simulink model "Sim_Induct_Harmon"  (R2017b)
settings: Solver=FixedStepAuto  StartTime=0.0  StopTime=t_total  FixedStep=1e-6  MaxStep=1e-4  RelTol=1e-3
values from neighbouring files (symbols this model uses):
  C21 = 100e-6    (= 0.0001)    [main_simu.m]
  C22 = 100e-6    (= 0.0001)    [main_simu.m]
  C23 = 220e-6    (= 0.00022)    [main_simu.m]
  C24 = 330e-6    (= 0.00033)    [main_simu.m]
  L41 = 10e-3    (= 0.01)    [main_simu.m]
  L42 = 10e-3    (= 0.01)    [main_simu.m]
  L43 = 10e-3    (= 0.01)    [main_simu.m]
  L44 = 100e-3    (= 0.1)    [main_simu.m]
  L61 = 1e-3    (= 0.001)    [main_simu.m]
  L62 = 1e-3    (= 0.001)    [main_simu.m]
  L63 = 1e-3    (= 0.001)    [main_simu.m]
  L64 = 1e-3    (= 0.001)    [main_simu.m]
  R21 = 2e3    (= 2000)    [main_simu.m]
  R22 = 1e3    (= 1000)    [main_simu.m]
  R23 = 500    [main_simu.m]
  R24 = 300    [main_simu.m]
  R31 = 2.5    [main_simu.m]
  R32 = 5    [main_simu.m]
  R33 = 8    [main_simu.m]
  R34 = 10    [main_simu.m]
  R41 = 10    [main_simu.m]
  R42 = 20    [main_simu.m]
  R43 = 30    [main_simu.m]
  R44 = 30    [main_simu.m]
  R51 = 10    [main_simu.m]
  R52 = 12    [main_simu.m]
  R53 = 15    [main_simu.m]
  R54 = 20    [main_simu.m]
  R61 = 10    [main_simu.m]
  R62 = 5    [main_simu.m]
  R63 = 30    [main_simu.m]
  R64 = 105    [main_simu.m]
  R71 = 5    [main_simu.m]
  R72 = 10    [main_simu.m]
  R73 = 20    [main_simu.m]
  R74 = 50    [main_simu.m]
  sim_off = sim_on    [double.m]    (also in fourfold.m; individual.m; main_simu.m; quintuple.m)
  sim_on = 50*ones(1,28)    [double.m]    (also in fourfold.m; individual.m; main_simu.m = 50*ones(1,num_cargas); quintuple.m)
  Valpha5 = 60    [main_simu.m]
  Valpha6 = 60    [main_simu.m]
undefined symbols (not defined in the file or in its folder): J, Laq, Lse, R, Ra, Rse, SEIP4, SEVP4, wm0, wmo
libraries: powerlib x225, simulink x72
(part 2 of 3)

== system Sim_Induct_Harmon/ON_OFF_25 ==
  Clock8 : Clock
  Compare To Constant5 : simulink/Logic and Bit Operations/Compare To Constant  relop=>=  const=sim_on(25)  OutDataTypeStr=boolean
  Compare To Constat6 : simulink/Logic and Bit Operations/Compare To Constant  relop=<=  const=sim_off(25)  OutDataTypeStr=boolean
  OFF5 : powerlib/Power Electronics/Ideal Switch  Ron=0.001  Lon=0  IC=0  Rs=1e5  Cs=inf  Measurements=off
  ON5 : powerlib/Power Electronics/Ideal Switch  Ron=0.001  Lon=0  IC=0  Rs=1e5  Cs=inf  Measurements=off
  Conn1 : PMIOPort  Port=1  Side=Left
  Conn2 : PMIOPort  Port=2  Side=Right
  wires:
  Clock8/1 -> Compare To Constat6/1, Compare To Constant5/1
  Compare To Constat6/1 -> OFF5/1
  Compare To Constant5/1 -> ON5/1
  connections:
  ON5/RConn1 -- OFF5/LConn1
  OFF5/RConn1 -- Conn2/RConn1
  ON5/LConn1 -- Conn1/RConn1

== system Sim_Induct_Harmon/ON_OFF_26 ==
  Clock8 : Clock
  Compare To Constant5 : simulink/Logic and Bit Operations/Compare To Constant  relop=>=  const=sim_on(26)  OutDataTypeStr=boolean
  Compare To Constat6 : simulink/Logic and Bit Operations/Compare To Constant  relop=<=  const=sim_off(26)  OutDataTypeStr=boolean
  OFF5 : powerlib/Power Electronics/Ideal Switch  Ron=0.001  Lon=0  IC=0  Rs=1e5  Cs=inf  Measurements=off
  ON5 : powerlib/Power Electronics/Ideal Switch  Ron=0.001  Lon=0  IC=0  Rs=1e5  Cs=inf  Measurements=off
  Conn1 : PMIOPort  Port=1  Side=Left
  Conn2 : PMIOPort  Port=2  Side=Right
  wires:
  Clock8/1 -> Compare To Constat6/1, Compare To Constant5/1
  Compare To Constat6/1 -> OFF5/1
  Compare To Constant5/1 -> ON5/1
  connections:
  ON5/RConn1 -- OFF5/LConn1
  OFF5/RConn1 -- Conn2/RConn1
  ON5/LConn1 -- Conn1/RConn1

== system Sim_Induct_Harmon/ON_OFF_27 ==
  Clock8 : Clock
  Compare To Constant5 : simulink/Logic and Bit Operations/Compare To Constant  relop=>=  const=sim_on(27)  OutDataTypeStr=boolean
  Compare To Constat6 : simulink/Logic and Bit Operations/Compare To Constant  relop=<=  const=sim_off(27)  OutDataTypeStr=boolean
  OFF5 : powerlib/Power Electronics/Ideal Switch  Ron=0.001  Lon=0  IC=0  Rs=1e5  Cs=inf  Measurements=off
  ON5 : powerlib/Power Electronics/Ideal Switch  Ron=0.001  Lon=0  IC=0  Rs=1e5  Cs=inf  Measurements=off
  Conn1 : PMIOPort  Port=1  Side=Left
  Conn2 : PMIOPort  Port=2  Side=Right
  wires:
  Clock8/1 -> Compare To Constat6/1, Compare To Constant5/1
  Compare To Constat6/1 -> OFF5/1
  Compare To Constant5/1 -> ON5/1
  connections:
  ON5/RConn1 -- OFF5/LConn1
  OFF5/RConn1 -- Conn2/RConn1
  ON5/LConn1 -- Conn1/RConn1

== system Sim_Induct_Harmon/ON_OFF_28 ==
  Clock8 : Clock
  Compare To Constant5 : simulink/Logic and Bit Operations/Compare To Constant  relop=>=  const=sim_on(28)  OutDataTypeStr=boolean
  Compare To Constat6 : simulink/Logic and Bit Operations/Compare To Constant  relop=<=  const=sim_off(28)  OutDataTypeStr=boolean
  OFF5 : powerlib/Power Electronics/Ideal Switch  Ron=0.001  Lon=0  IC=0  Rs=1e5  Cs=inf  Measurements=off
  ON5 : powerlib/Power Electronics/Ideal Switch  Ron=0.001  Lon=0  IC=0  Rs=1e5  Cs=inf  Measurements=off
  Conn1 : PMIOPort  Port=1  Side=Left
  Conn2 : PMIOPort  Port=2  Side=Right
  wires:
  Clock8/1 -> Compare To Constat6/1, Compare To Constant5/1
  Compare To Constat6/1 -> OFF5/1
  Compare To Constant5/1 -> ON5/1
  connections:
  ON5/RConn1 -- OFF5/LConn1
  OFF5/RConn1 -- Conn2/RConn1
  ON5/LConn1 -- Conn1/RConn1

== system Sim_Induct_Harmon/ON_OFF_3 ==
  Clock1 : Clock
  Clock2 : Clock
  Clock3 : Clock
  Compare To Constant : simulink/Logic and Bit Operations/Compare To Constant  relop=>=  const=sim_on(3)  OutDataTypeStr=boolean
  Compare To Constant1 : simulink/Logic and Bit Operations/Compare To Constant  relop=>=  const=sim_off(3)  OutDataTypeStr=boolean
  Compare To Constant2 : simulink/Logic and Bit Operations/Compare To Constant  relop=>=  const=sim_on(3)  OutDataTypeStr=boolean
  Constant : Constant  Value=0
  Constant1 : Constant  Value=0
  Ideal Switch : powerlib/Power Electronics/Ideal Switch  Ron=0.001  Lon=0  IC=0  Rs=1e5  Cs=inf  Measurements=off
  Switch : Switch
  Switch1 : Switch
  Conn1 : PMIOPort  Port=1  Side=Left
  Conn2 : PMIOPort  Port=2  Side=Left
  tag scope: tensao_3=global
  wires:
  Switch1/1 -> [tensao_3]
  Constant/1 -> Switch/3
  Switch/1 -> Switch1/3
  Clock1/1 -> Compare To Constant/1
  Clock2/1 -> Compare To Constant1/1
  Compare To Constant1/1 -> Switch1/2
  [fonte_tensao] -> Switch/1
  Constant1/1 -> Switch1/1
  Compare To Constant/1 -> Switch/2
  Clock3/1 -> Compare To Constant2/1
  Compare To Constant2/1 -> Ideal Switch/1
  connections:
  Conn1/RConn1 -- Ideal Switch/LConn1
  Ideal Switch/RConn1 -- Conn2/RConn1

== system Sim_Induct_Harmon/ON_OFF_4 ==
  Clock1 : Clock
  Clock2 : Clock
  Clock3 : Clock
  Compare To Constant : simulink/Logic and Bit Operations/Compare To Constant  relop=>=  const=sim_on(4)  OutDataTypeStr=boolean
  Compare To Constant1 : simulink/Logic and Bit Operations/Compare To Constant  relop=>=  const=sim_off(4)  OutDataTypeStr=boolean
  Compare To Constant2 : simulink/Logic and Bit Operations/Compare To Constant  relop=>=  const=sim_on(4)  OutDataTypeStr=boolean
  Constant : Constant  Value=0
  Constant1 : Constant  Value=0
  Ideal Switch : powerlib/Power Electronics/Ideal Switch  Ron=0.001  Lon=0  IC=0  Rs=1e5  Cs=inf  Measurements=off
  Switch : Switch
  Switch1 : Switch
  Conn1 : PMIOPort  Port=1  Side=Left
  Conn2 : PMIOPort  Port=2  Side=Left
  tag scope: tensao_4=global
  wires:
  Switch1/1 -> [tensao_4]
  Constant/1 -> Switch/3
  Switch/1 -> Switch1/3
  Clock1/1 -> Compare To Constant/1
  Clock2/1 -> Compare To Constant1/1
  Compare To Constant1/1 -> Switch1/2
  [fonte_tensao] -> Switch/1
  Constant1/1 -> Switch1/1
  Compare To Constant/1 -> Switch/2
  Clock3/1 -> Compare To Constant2/1
  Compare To Constant2/1 -> Ideal Switch/1
  connections:
  Conn1/RConn1 -- Ideal Switch/LConn1
  Ideal Switch/RConn1 -- Conn2/RConn1

== system Sim_Induct_Harmon/ON_OFF_5 ==
  Clock1 : Clock
  Compare To Constant1 : simulink/Logic and Bit Operations/Compare To Constant  relop=>=  const=sim_on(5)  OutDataTypeStr=boolean
  Compare To Constat1 : simulink/Logic and Bit Operations/Compare To Constant  relop=<=  const=sim_off(5)  OutDataTypeStr=boolean
  OFF1 : powerlib/Power Electronics/Ideal Switch  Ron=0.001  Lon=0  IC=0  Rs=1e5  Cs=inf  Measurements=off
  ON1 : powerlib/Power Electronics/Ideal Switch  Ron=0.001  Lon=0  IC=0  Rs=1e5  Cs=inf  Measurements=off
  Conn1 : PMIOPort  Port=1  Side=Left
  Conn2 : PMIOPort  Port=2  Side=Right
  wires:
  Compare To Constat1/1 -> OFF1/1
  Compare To Constant1/1 -> ON1/1
  Clock1/1 -> Compare To Constat1/1, Compare To Constant1/1
  connections:
  ON1/RConn1 -- OFF1/LConn1
  Conn1/RConn1 -- ON1/LConn1
  OFF1/RConn1 -- Conn2/RConn1

== system Sim_Induct_Harmon/ON_OFF_6 ==
  Clock1 : Clock
  Compare To Constant1 : simulink/Logic and Bit Operations/Compare To Constant  relop=>=  const=sim_on(6)  OutDataTypeStr=boolean
  Compare To Constat1 : simulink/Logic and Bit Operations/Compare To Constant  relop=<=  const=sim_off(6)  OutDataTypeStr=boolean
  OFF1 : powerlib/Power Electronics/Ideal Switch  Ron=0.001  Lon=0  IC=0  Rs=1e5  Cs=inf  Measurements=off
  ON1 : powerlib/Power Electronics/Ideal Switch  Ron=0.001  Lon=0  IC=0  Rs=1e5  Cs=inf  Measurements=off
  Conn1 : PMIOPort  Port=1  Side=Left
  Conn2 : PMIOPort  Port=2  Side=Right
  wires:
  Compare To Constat1/1 -> OFF1/1
  Compare To Constant1/1 -> ON1/1
  Clock1/1 -> Compare To Constat1/1, Compare To Constant1/1
  connections:
  ON1/RConn1 -- OFF1/LConn1
  Conn1/RConn1 -- ON1/LConn1
  OFF1/RConn1 -- Conn2/RConn1

== system Sim_Induct_Harmon/ON_OFF_7 ==
  Clock1 : Clock
  Compare To Constant1 : simulink/Logic and Bit Operations/Compare To Constant  relop=>=  const=sim_on(7)  OutDataTypeStr=boolean
  Compare To Constat1 : simulink/Logic and Bit Operations/Compare To Constant  relop=<=  const=sim_off(7)  OutDataTypeStr=boolean
  OFF1 : powerlib/Power Electronics/Ideal Switch  Ron=0.001  Lon=0  IC=0  Rs=1e5  Cs=inf  Measurements=off
  ON1 : powerlib/Power Electronics/Ideal Switch  Ron=0.001  Lon=0  IC=0  Rs=1e5  Cs=inf  Measurements=off
  Conn1 : PMIOPort  Port=1  Side=Left
  Conn2 : PMIOPort  Port=2  Side=Right
  wires:
  Compare To Constat1/1 -> OFF1/1
  Compare To Constant1/1 -> ON1/1
  Clock1/1 -> Compare To Constat1/1, Compare To Constant1/1
  connections:
  ON1/RConn1 -- OFF1/LConn1
  Conn1/RConn1 -- ON1/LConn1
  OFF1/RConn1 -- Conn2/RConn1

== system Sim_Induct_Harmon/ON_OFF_8 ==
  Clock1 : Clock
  Compare To Constant1 : simulink/Logic and Bit Operations/Compare To Constant  relop=>=  const=sim_on(8)  OutDataTypeStr=boolean
  Compare To Constat1 : simulink/Logic and Bit Operations/Compare To Constant  relop=<=  const=sim_off(8)  OutDataTypeStr=boolean
  OFF1 : powerlib/Power Electronics/Ideal Switch  Ron=0.001  Lon=0  IC=0  Rs=1e5  Cs=inf  Measurements=off
  ON1 : powerlib/Power Electronics/Ideal Switch  Ron=0.001  Lon=0  IC=0  Rs=1e5  Cs=inf  Measurements=off
  Conn1 : PMIOPort  Port=1  Side=Left
  Conn2 : PMIOPort  Port=2  Side=Right
  wires:
  Compare To Constat1/1 -> OFF1/1
  Compare To Constant1/1 -> ON1/1
  Clock1/1 -> Compare To Constat1/1, Compare To Constant1/1
  connections:
  ON1/RConn1 -- OFF1/LConn1
  Conn1/RConn1 -- ON1/LConn1
  OFF1/RConn1 -- Conn2/RConn1

== system Sim_Induct_Harmon/ON_OFF_9 ==
  Clock4 : Clock
  Compare To Constant2 : simulink/Logic and Bit Operations/Compare To Constant  relop=>=  const=sim_on(9)  OutDataTypeStr=boolean
  Compare To Constat3 : simulink/Logic and Bit Operations/Compare To Constant  relop=<=  const=sim_off(9)  OutDataTypeStr=boolean
  OFF2 : powerlib/Power Electronics/Ideal Switch  Ron=0.001  Lon=0  IC=0  Rs=1e5  Cs=inf  Measurements=off
  ON2 : powerlib/Power Electronics/Ideal Switch  Ron=0.001  Lon=0  IC=0  Rs=1e5  Cs=inf  Measurements=off
  Conn1 : PMIOPort  Port=1  Side=Left
  Conn2 : PMIOPort  Port=2  Side=Right
  wires:
  Compare To Constant2/1 -> ON2/1
  Compare To Constat3/1 -> OFF2/1
  Clock4/1 -> Compare To Constat3/1, Compare To Constant2/1
  connections:
  OFF2/RConn1 -- Conn2/RConn1
  ON2/RConn1 -- OFF2/LConn1
  ON2/LConn1 -- Conn1/RConn1

== system Sim_Induct_Harmon/PONTE_DIODO_1 ==
  Diode{,1..3} (4 alike) : powerlib/Power Electronics/Diode  Ron=0.001  Lon=0  Vf=0.8  IC=0  UseSnubber=0  Rs=500  Cs=250e-9  Measurements=off
  Scope : Scope
  Scope1 : Scope
  Series RLC Branch : powerlib/Elements/Series RLC Branch  LConnTagsString=__new0  RConnTagsString=__new0  BranchType=C  Resistance=R  Inductance=1e-3  SetiL0=off  InitialCurrent=0  Capacitance=C21  Setx0=off  InitialVoltage=0  Measurements=None
  Series RLC Branch1 : powerlib/Elements/Series RLC Branch  LConnTagsString=__new0  RConnTagsString=__new0  BranchType=R  Resistance=R21  Inductance=1e-3  SetiL0=off  InitialCurrent=0  Capacitance=1e-6  Setx0=off  InitialVoltage=0  Measurements=None
  Series RLC Branch2 : powerlib/Elements/Series RLC Branch  LConnTagsString=__new0  RConnTagsString=__new0  BranchType=R  Resistance=10  Inductance=1e-3  SetiL0=off  InitialCurrent=0  Capacitance=C21  Setx0=off  InitialVoltage=0  Measurements=None
  To Workspace1 : ToWorkspace  VariableName=corrente_ponte_1  SampleTime=-1
  To Workspace4 : ToWorkspace  VariableName=tensao_ponte_1  SampleTime=-1
  V_Load : powerlib/Measurements/Voltage Measurement  PhasorSimulation=off  OutputType=Complex  PSBequivalent=0
  i_Load : powerlib/Measurements/Current Measurement  Tag=PoWeRsYsTeMmEaSuReMeNt  PhasorSimulation=off  OutputType=Magnitude  PSBequivalent=0
  Conn1 : PMIOPort  Port=1  Side=Left
  Conn2 : PMIOPort  Port=2  Side=Left
  wires:
  i_Load/1 -> To Workspace1/1, Scope1/1
  V_Load/1 -> To Workspace4/1, Scope/1
  connections:
  Conn1/RConn1 -- i_Load/LConn1
  Diode1/LConn1 -- Conn2/RConn1 -- Diode3/RConn1
  Series RLC Branch/LConn1 -- Diode/RConn1 -- Diode1/RConn1 -- V_Load/LConn1 -- Series RLC Branch1/LConn1
  Series RLC Branch/RConn1 -- Diode2/LConn1 -- Diode3/LConn1 -- V_Load/LConn2 -- Series RLC Branch1/RConn1
  Series RLC Branch2/RConn1 -- Diode2/RConn1 -- Diode/LConn1
  i_Load/RConn1 -- Series RLC Branch2/LConn1

== system Sim_Induct_Harmon/PONTE_DIODO_2 ==
  Diode{,1..3} (4 alike) : powerlib/Power Electronics/Diode  Ron=0.001  Lon=0  Vf=0.8  IC=0  UseSnubber=0  Rs=500  Cs=250e-9  Measurements=off
  Scope : Scope
  Scope1 : Scope
  Series RLC Branch : powerlib/Elements/Series RLC Branch  LConnTagsString=__new0  RConnTagsString=__new0  BranchType=C  Resistance=R  Inductance=1e-3  SetiL0=off  InitialCurrent=0  Capacitance=C22  Setx0=off  InitialVoltage=0  Measurements=None
  Series RLC Branch1 : powerlib/Elements/Series RLC Branch  LConnTagsString=__new0  RConnTagsString=__new0  BranchType=R  Resistance=R22  Inductance=1e-3  SetiL0=off  InitialCurrent=0  Capacitance=1e-6  Setx0=off  InitialVoltage=0  Measurements=None
  Series RLC Branch2 : powerlib/Elements/Series RLC Branch  LConnTagsString=__new0  RConnTagsString=__new0  BranchType=R  Resistance=10  Inductance=1e-3  SetiL0=off  InitialCurrent=0  Capacitance=C21  Setx0=off  InitialVoltage=0  Measurements=None
  To Workspace1 : ToWorkspace  VariableName=corrente_ponte_2  SampleTime=-1
  To Workspace4 : ToWorkspace  VariableName=tensao_ponte_2  SampleTime=-1
  V_Load : powerlib/Measurements/Voltage Measurement  PhasorSimulation=off  OutputType=Complex  PSBequivalent=0
  i_Load : powerlib/Measurements/Current Measurement  Tag=PoWeRsYsTeMmEaSuReMeNt  PhasorSimulation=off  OutputType=Magnitude  PSBequivalent=0
  Conn1 : PMIOPort  Port=1  Side=Left
  Conn2 : PMIOPort  Port=2  Side=Left
  wires:
  i_Load/1 -> To Workspace1/1, Scope1/1
  V_Load/1 -> To Workspace4/1, Scope/1
  connections:
  Conn1/RConn1 -- i_Load/LConn1
  Diode1/LConn1 -- Conn2/RConn1 -- Diode3/RConn1
  Series RLC Branch/LConn1 -- Diode/RConn1 -- Diode1/RConn1 -- V_Load/LConn1 -- Series RLC Branch1/LConn1
  Series RLC Branch/RConn1 -- Diode2/LConn1 -- Diode3/LConn1 -- V_Load/LConn2 -- Series RLC Branch1/RConn1
  Diode2/RConn1 -- Series RLC Branch2/RConn1 -- Diode/LConn1
  i_Load/RConn1 -- Series RLC Branch2/LConn1

== system Sim_Induct_Harmon/PONTE_DIODO_3 ==
  Diode{,1..3} (4 alike) : powerlib/Power Electronics/Diode  Ron=0.001  Lon=0  Vf=0.8  IC=0  UseSnubber=0  Rs=500  Cs=250e-9  Measurements=off
  Scope : Scope
  Scope1 : Scope
  Series RLC Branch : powerlib/Elements/Series RLC Branch  LConnTagsString=__new0  RConnTagsString=__new0  BranchType=C  Resistance=R  Inductance=1e-3  SetiL0=off  InitialCurrent=0  Capacitance=C23  Setx0=off  InitialVoltage=0  Measurements=None
  Series RLC Branch1 : powerlib/Elements/Series RLC Branch  LConnTagsString=__new0  RConnTagsString=__new0  BranchType=R  Resistance=R23  Inductance=1e-3  SetiL0=off  InitialCurrent=0  Capacitance=1e-6  Setx0=off  InitialVoltage=0  Measurements=None
  Series RLC Branch2 : powerlib/Elements/Series RLC Branch  LConnTagsString=__new0  RConnTagsString=__new0  BranchType=R  Resistance=10  Inductance=1e-3  SetiL0=off  InitialCurrent=0  Capacitance=C21  Setx0=off  InitialVoltage=0  Measurements=None
  To Workspace1 : ToWorkspace  VariableName=corrente_ponte_3  SampleTime=-1
  To Workspace4 : ToWorkspace  VariableName=tensao_ponte_3  SampleTime=-1
  V_Load : powerlib/Measurements/Voltage Measurement  PhasorSimulation=off  OutputType=Complex  PSBequivalent=0
  i_Load : powerlib/Measurements/Current Measurement  Tag=PoWeRsYsTeMmEaSuReMeNt  PhasorSimulation=off  OutputType=Magnitude  PSBequivalent=0
  powergui : powerlib/powergui  Priority=1  SimulationMode=Discrete  SampleTime=1e-6  frequency=60  Iterations=100  frequencyindice=60  Pbase=100e6  ErrMax=1e-4  UnitsV=kV  UnitsW=MW  buscounter=0  FunctionMessages=off  echomessages=off  EnableUseOfTLC=off  CurrentSourceSwitches=off  DisableSnubberDevices=off  DisableRonSwitches=off  DisableVfSwitches=off  DisplayEquations=off  SolverType=Tustin/Backward Euler (TBE)  Interpol=off  ExternalGateDelay=off  methode=off  Ts=100  x0status=zero  SPID=off  SwTol=0  HookPort=off  RestoreLinks=warning  ResistiveCurrentMeasurement=off  Frange=[0:2:500]  Ylog=off  Xlog=on  ShowGrid=off  save=off  variable=ZData  structure=0  ZoomFFT=off  StartTime=0.0  cycles=1  DisplayStyle=1  fundamental=60  FreqAxis=off  MaxFrequency=1000  frequencyindicesteady=1  RmsSteady=1  display=off
  Conn1 : PMIOPort  Port=1  Side=Left
  Conn2 : PMIOPort  Port=2  Side=Left
  wires:
  i_Load/1 -> To Workspace1/1, Scope1/1
  V_Load/1 -> To Workspace4/1, Scope/1
  connections:
  Conn1/RConn1 -- i_Load/LConn1
  Diode1/LConn1 -- Conn2/RConn1 -- Diode3/RConn1
  Series RLC Branch/LConn1 -- Diode/RConn1 -- Diode1/RConn1 -- V_Load/LConn1 -- Series RLC Branch1/LConn1
  Series RLC Branch/RConn1 -- Diode2/LConn1 -- Diode3/LConn1 -- V_Load/LConn2 -- Series RLC Branch1/RConn1
  Diode/LConn1 -- Series RLC Branch2/RConn1 -- Diode2/RConn1
  i_Load/RConn1 -- Series RLC Branch2/LConn1

== system Sim_Induct_Harmon/PONTE_DIODO_4 ==
  Diode{,1..3} (4 alike) : powerlib/Power Electronics/Diode  Ron=0.001  Lon=0  Vf=0.8  IC=0  UseSnubber=0  Rs=500  Cs=250e-9  Measurements=off
  Scope : Scope
  Scope1 : Scope
  Series RLC Branch : powerlib/Elements/Series RLC Branch  LConnTagsString=__new0  RConnTagsString=__new0  BranchType=C  Resistance=R  Inductance=1e-3  SetiL0=off  InitialCurrent=0  Capacitance=C24  Setx0=off  InitialVoltage=0  Measurements=None
  Series RLC Branch1 : powerlib/Elements/Series RLC Branch  LConnTagsString=__new0  RConnTagsString=__new0  BranchType=R  Resistance=R24  Inductance=1e-3  SetiL0=off  InitialCurrent=0  Capacitance=1e-6  Setx0=off  InitialVoltage=0  Measurements=None
  Series RLC Branch2 : powerlib/Elements/Series RLC Branch  LConnTagsString=__new0  RConnTagsString=__new0  BranchType=R  Resistance=10  Inductance=1e-3  SetiL0=off  InitialCurrent=0  Capacitance=C21  Setx0=off  InitialVoltage=0  Measurements=None
  To Workspace1 : ToWorkspace  VariableName=corrente_ponte_4  SampleTime=-1
  To Workspace4 : ToWorkspace  VariableName=tensao_ponte_4  SampleTime=-1
  V_Load : powerlib/Measurements/Voltage Measurement  PhasorSimulation=off  OutputType=Complex  PSBequivalent=0
  i_Load : powerlib/Measurements/Current Measurement  Tag=PoWeRsYsTeMmEaSuReMeNt  PhasorSimulation=off  OutputType=Magnitude  PSBequivalent=0
  Conn1 : PMIOPort  Port=1  Side=Left
  Conn2 : PMIOPort  Port=2  Side=Left
  wires:
  i_Load/1 -> To Workspace1/1, Scope1/1
  V_Load/1 -> To Workspace4/1, Scope/1
  connections:
  Conn1/RConn1 -- i_Load/LConn1
  Diode1/LConn1 -- Conn2/RConn1 -- Diode3/RConn1
  Series RLC Branch/LConn1 -- Diode/RConn1 -- Diode1/RConn1 -- V_Load/LConn1 -- Series RLC Branch1/LConn1
  Series RLC Branch/RConn1 -- Diode2/LConn1 -- Diode3/LConn1 -- V_Load/LConn2 -- Series RLC Branch1/RConn1
  Diode/LConn1 -- Series RLC Branch2/RConn1 -- Diode2/RConn1
  i_Load/RConn1 -- Series RLC Branch2/LConn1

== system Sim_Induct_Harmon/RL_1 ==
  note: LOAD
  Scope : Scope
  Scope1 : Scope
  Series RLC Branch : powerlib/Elements/Series RLC Branch  LConnTagsString=__new0  RConnTagsString=__new0  BranchType=R  Resistance=R41  Inductance=1e-3  SetiL0=off  InitialCurrent=0  Capacitance=1e-6  Setx0=off  InitialVoltage=0  Measurements=None
  Series RLC Branch1 : powerlib/Elements/Series RLC Branch  LConnTagsString=__new0  RConnTagsString=__new0  BranchType=L  Resistance=1  Inductance=L41  SetiL0=off  InitialCurrent=0  Capacitance=1e-6  Setx0=off  InitialVoltage=0  Measurements=None
  To Workspace1 : ToWorkspace  VariableName=corrente_rl_1  SampleTime=-1
  To Workspace4 : ToWorkspace  VariableName=tensao_rl_1  SampleTime=-1
  V_Load : powerlib/Measurements/Voltage Measurement  PhasorSimulation=off  OutputType=Complex  PSBequivalent=0
  i_Load : powerlib/Measurements/Current Measurement  Tag=PoWeRsYsTeMmEaSuReMeNt  PhasorSimulation=off  OutputType=Magnitude  PSBequivalent=0
  Conn1 : PMIOPort  Port=1  Side=Left
  Conn2 : PMIOPort  Port=2  Side=Left
  wires:
  V_Load/1 -> To Workspace4/1, Scope/1
  i_Load/1 -> To Workspace1/1, Scope1/1
  connections:
  Series RLC Branch/LConn1 -- V_Load/LConn1 -- i_Load/RConn1
  Conn1/RConn1 -- i_Load/LConn1
  V_Load/LConn2 -- Conn2/RConn1 -- Series RLC Branch1/RConn1
  Series RLC Branch1/LConn1 -- Series RLC Branch/RConn1

== system Sim_Induct_Harmon/RL_2 ==
  note: LOAD
  Scope : Scope
  Scope1 : Scope
  Series RLC Branch : powerlib/Elements/Series RLC Branch  LConnTagsString=__new0  RConnTagsString=__new0  BranchType=R  Resistance=R42  Inductance=1e-3  SetiL0=off  InitialCurrent=0  Capacitance=1e-6  Setx0=off  InitialVoltage=0  Measurements=None
  Series RLC Branch1 : powerlib/Elements/Series RLC Branch  LConnTagsString=__new0  RConnTagsString=__new0  BranchType=L  Resistance=1  Inductance=L42  SetiL0=off  InitialCurrent=0  Capacitance=1e-6  Setx0=off  InitialVoltage=0  Measurements=None
  To Workspace1 : ToWorkspace  VariableName=corrente_rl_2  SampleTime=-1
  To Workspace4 : ToWorkspace  VariableName=tensao_rl_2  SampleTime=-1
  V_Load : powerlib/Measurements/Voltage Measurement  PhasorSimulation=off  OutputType=Complex  PSBequivalent=0
  i_Load : powerlib/Measurements/Current Measurement  Tag=PoWeRsYsTeMmEaSuReMeNt  PhasorSimulation=off  OutputType=Magnitude  PSBequivalent=0
  Conn1 : PMIOPort  Port=1  Side=Left
  Conn2 : PMIOPort  Port=2  Side=Left
  wires:
  V_Load/1 -> To Workspace4/1, Scope/1
  i_Load/1 -> To Workspace1/1, Scope1/1
  connections:
  Series RLC Branch/LConn1 -- V_Load/LConn1 -- i_Load/RConn1
  Conn1/RConn1 -- i_Load/LConn1
  V_Load/LConn2 -- Conn2/RConn1 -- Series RLC Branch1/RConn1
  Series RLC Branch1/LConn1 -- Series RLC Branch/RConn1

== system Sim_Induct_Harmon/RL_3 ==
  note: LOAD
  Scope : Scope
  Scope1 : Scope
  Series RLC Branch : powerlib/Elements/Series RLC Branch  LConnTagsString=__new0  RConnTagsString=__new0  BranchType=R  Resistance=R43  Inductance=1e-3  SetiL0=off  InitialCurrent=0  Capacitance=1e-6  Setx0=off  InitialVoltage=0  Measurements=None
  Series RLC Branch1 : powerlib/Elements/Series RLC Branch  LConnTagsString=__new0  RConnTagsString=__new0  BranchType=L  Resistance=1  Inductance=L43  SetiL0=off  InitialCurrent=0  Capacitance=1e-6  Setx0=off  InitialVoltage=0  Measurements=None
  To Workspace1 : ToWorkspace  VariableName=corrente_rl_3  SampleTime=-1
  To Workspace4 : ToWorkspace  VariableName=tensao_rl_3  SampleTime=-1
  V_Load : powerlib/Measurements/Voltage Measurement  PhasorSimulation=off  OutputType=Complex  PSBequivalent=0
  i_Load : powerlib/Measurements/Current Measurement  Tag=PoWeRsYsTeMmEaSuReMeNt  PhasorSimulation=off  OutputType=Magnitude  PSBequivalent=0
  Conn1 : PMIOPort  Port=1  Side=Left
  Conn2 : PMIOPort  Port=2  Side=Left
  wires:
  V_Load/1 -> To Workspace4/1, Scope/1
  i_Load/1 -> To Workspace1/1, Scope1/1
  connections:
  Series RLC Branch/LConn1 -- V_Load/LConn1 -- i_Load/RConn1
  Conn1/RConn1 -- i_Load/LConn1
  V_Load/LConn2 -- Conn2/RConn1 -- Series RLC Branch1/RConn1
  Series RLC Branch1/LConn1 -- Series RLC Branch/RConn1

== system Sim_Induct_Harmon/RL_4 ==
  note: LOAD
  Scope : Scope
  Scope1 : Scope
  Series RLC Branch : powerlib/Elements/Series RLC Branch  LConnTagsString=__new0  RConnTagsString=__new0  BranchType=R  Resistance=R44  Inductance=1e-3  SetiL0=off  InitialCurrent=0  Capacitance=1e-6  Setx0=off  InitialVoltage=0  Measurements=None
  Series RLC Branch1 : powerlib/Elements/Series RLC Branch  LConnTagsString=__new0  RConnTagsString=__new0  BranchType=L  Resistance=1  Inductance=L44  SetiL0=off  InitialCurrent=0  Capacitance=1e-6  Setx0=off  InitialVoltage=0  Measurements=None
  To Workspace1 : ToWorkspace  VariableName=corrente_rl_4  SampleTime=-1
  To Workspace4 : ToWorkspace  VariableName=tensao_rl_4  SampleTime=-1
  V_Load : powerlib/Measurements/Voltage Measurement  PhasorSimulation=off  OutputType=Complex  PSBequivalent=0
  i_Load : powerlib/Measurements/Current Measurement  Tag=PoWeRsYsTeMmEaSuReMeNt  PhasorSimulation=off  OutputType=Magnitude  PSBequivalent=0
  Conn1 : PMIOPort  Port=1  Side=Left
  Conn2 : PMIOPort  Port=2  Side=Left
  wires:
  V_Load/1 -> To Workspace4/1, Scope/1
  i_Load/1 -> To Workspace1/1, Scope1/1
  connections:
  Series RLC Branch/LConn1 -- V_Load/LConn1 -- i_Load/RConn1
  Conn1/RConn1 -- i_Load/LConn1
  V_Load/LConn2 -- Conn2/RConn1 -- Series RLC Branch1/RConn1
  Series RLC Branch1/LConn1 -- Series RLC Branch/RConn1

== system Sim_Induct_Harmon/R_1 ==
  note: LOAD
  Scope : Scope
  Scope1 : Scope
  Series RLC Branch : powerlib/Elements/Series RLC Branch  LConnTagsString=__new0  RConnTagsString=__new0  BranchType=R  Resistance=R31  Inductance=1e-3  SetiL0=off  InitialCurrent=0  Capacitance=1e-6  Setx0=off  InitialVoltage=0  Measurements=None
  To Workspace1 : ToWorkspace  VariableName=corrente_r_1  SampleTime=-1
  To Workspace4 : ToWorkspace  VariableName=tensao_r_1  SampleTime=-1
  V_Load : powerlib/Measurements/Voltage Measurement  PhasorSimulation=off  OutputType=Complex  PSBequivalent=0
  i_Load : powerlib/Measurements/Current Measurement  Tag=PoWeRsYsTeMmEaSuReMeNt  PhasorSimulation=off  OutputType=Magnitude  PSBequivalent=0
  Conn1 : PMIOPort  Port=1  Side=Left
  Conn2 : PMIOPort  Port=2  Side=Left
  wires:
  V_Load/1 -> To Workspace4/1, Scope/1
  i_Load/1 -> To Workspace1/1, Scope1/1
  connections:
  Series RLC Branch/LConn1 -- V_Load/LConn1 -- i_Load/RConn1
  Series RLC Branch/RConn1 -- V_Load/LConn2 -- Conn2/RConn1
  Conn1/RConn1 -- i_Load/LConn1

== system Sim_Induct_Harmon/R_2 ==
  note: LOAD
  Scope : Scope
  Scope1 : Scope
  Series RLC Branch : powerlib/Elements/Series RLC Branch  LConnTagsString=__new0  RConnTagsString=__new0  BranchType=R  Resistance=R32  Inductance=1e-3  SetiL0=off  InitialCurrent=0  Capacitance=1e-6  Setx0=off  InitialVoltage=0  Measurements=None
  To Workspace1 : ToWorkspace  VariableName=corrente_r_2  SampleTime=-1
  To Workspace4 : ToWorkspace  VariableName=tensao_r_2  SampleTime=-1
  V_Load : powerlib/Measurements/Voltage Measurement  PhasorSimulation=off  OutputType=Complex  PSBequivalent=0
  i_Load : powerlib/Measurements/Current Measurement  Tag=PoWeRsYsTeMmEaSuReMeNt  PhasorSimulation=off  OutputType=Magnitude  PSBequivalent=0
  Conn1 : PMIOPort  Port=1  Side=Left
  Conn2 : PMIOPort  Port=2  Side=Left
  wires:
  V_Load/1 -> To Workspace4/1, Scope/1
  i_Load/1 -> To Workspace1/1, Scope1/1
  connections:
  Series RLC Branch/LConn1 -- V_Load/LConn1 -- i_Load/RConn1
  Series RLC Branch/RConn1 -- V_Load/LConn2 -- Conn2/RConn1
  Conn1/RConn1 -- i_Load/LConn1

== system Sim_Induct_Harmon/R_3 ==
  note: LOAD
  Scope : Scope
  Scope1 : Scope
  Series RLC Branch : powerlib/Elements/Series RLC Branch  LConnTagsString=__new0  RConnTagsString=__new0  BranchType=R  Resistance=R33  Inductance=1e-3  SetiL0=off  InitialCurrent=0  Capacitance=1e-6  Setx0=off  InitialVoltage=0  Measurements=None
  To Workspace1 : ToWorkspace  VariableName=corrente_r_3  SampleTime=-1
  To Workspace4 : ToWorkspace  VariableName=tensao_r_3  SampleTime=-1
  V_Load : powerlib/Measurements/Voltage Measurement  PhasorSimulation=off  OutputType=Complex  PSBequivalent=0
  i_Load : powerlib/Measurements/Current Measurement  Tag=PoWeRsYsTeMmEaSuReMeNt  PhasorSimulation=off  OutputType=Magnitude  PSBequivalent=0
  Conn1 : PMIOPort  Port=1  Side=Left
  Conn2 : PMIOPort  Port=2  Side=Left
  wires:
  V_Load/1 -> To Workspace4/1, Scope/1
  i_Load/1 -> To Workspace1/1, Scope1/1
  connections:
  Series RLC Branch/LConn1 -- V_Load/LConn1 -- i_Load/RConn1
  Series RLC Branch/RConn1 -- V_Load/LConn2 -- Conn2/RConn1
  Conn1/RConn1 -- i_Load/LConn1

== system Sim_Induct_Harmon/R_4 ==
  note: LOAD
  Scope : Scope
  Scope1 : Scope
  Series RLC Branch : powerlib/Elements/Series RLC Branch  LConnTagsString=__new0  RConnTagsString=__new0  BranchType=R  Resistance=R34  Inductance=1e-3  SetiL0=off  InitialCurrent=0  Capacitance=1e-6  Setx0=off  InitialVoltage=0  Measurements=None
  To Workspace1 : ToWorkspace  VariableName=corrente_r_4  SampleTime=-1
  To Workspace4 : ToWorkspace  VariableName=tensao_r_4  SampleTime=-1
  V_Load : powerlib/Measurements/Voltage Measurement  PhasorSimulation=off  OutputType=Complex  PSBequivalent=0
  i_Load : powerlib/Measurements/Current Measurement  Tag=PoWeRsYsTeMmEaSuReMeNt  PhasorSimulation=off  OutputType=Magnitude  PSBequivalent=0
  Conn1 : PMIOPort  Port=1  Side=Left
  Conn2 : PMIOPort  Port=2  Side=Left
  wires:
  V_Load/1 -> To Workspace4/1, Scope/1
  i_Load/1 -> To Workspace1/1, Scope1/1
  connections:
  Series RLC Branch/LConn1 -- V_Load/LConn1 -- i_Load/RConn1
  Series RLC Branch/RConn1 -- V_Load/LConn2 -- Conn2/RConn1
  Conn1/RConn1 -- i_Load/LConn1

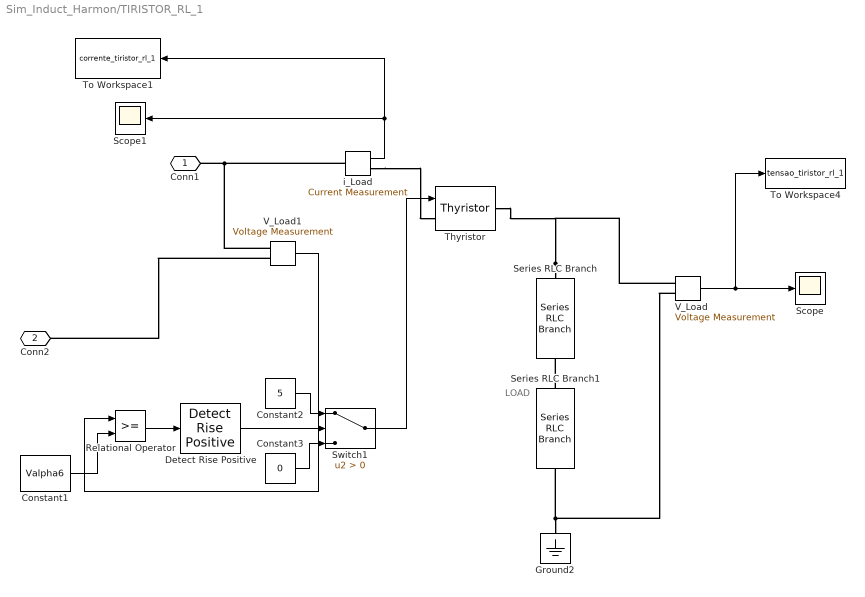
== system Sim_Induct_Harmon/TIRISTOR_RL_1 ==
  note: LOAD
  Constant1 : Constant  Value=Valpha6
  Constant2 : Constant  Value=5
  Constant3 : Constant  Value=0
  Detect Rise Positive : simulink/Logic and Bit Operations/Detect Rise Positive  vinit=0  OutDataTypeStr=boolean
  Ground2 : powerlib/Elements/Ground  LConnTagsString=a
  Relational Operator : RelationalOperator  OutDataTypeStr=boolean  RndMeth=Simplest
  Scope : Scope
  Scope1 : Scope
  Series RLC Branch : powerlib/Elements/Series RLC Branch  LConnTagsString=__new0  RConnTagsString=__new0  BranchType=R  Resistance=R61  Inductance=1e-3  SetiL0=off  InitialCurrent=0  Capacitance=1e-6  Setx0=off  InitialVoltage=0  Measurements=None
  Series RLC Branch1 : powerlib/Elements/Series RLC Branch  LConnTagsString=__new0  RConnTagsString=__new0  BranchType=L  Resistance=1  Inductance=L61  SetiL0=off  InitialCurrent=0  Capacitance=1e-6  Setx0=off  InitialVoltage=0  Measurements=None
  Switch1 : Switch  Criteria=u2 > Threshold
  Thyristor : powerlib/Power Electronics/Thyristor  Ron=0.001  Lon=0  Vf=0.8  IC=0  Rs=500  Cs=250e-9  Measurements=off
  To Workspace1 : ToWorkspace  VariableName=corrente_tiristor_rl_1  SampleTime=-1
  To Workspace4 : ToWorkspace  VariableName=tensao_tiristor_rl_1  SampleTime=-1
  V_Load : powerlib/Measurements/Voltage Measurement  PhasorSimulation=off  OutputType=Complex  PSBequivalent=0
  V_Load1 : powerlib/Measurements/Voltage Measurement  PhasorSimulation=off  OutputType=Complex  PSBequivalent=0
  i_Load : powerlib/Measurements/Current Measurement  Tag=PoWeRsYsTeMmEaSuReMeNt  PhasorSimulation=off  OutputType=Magnitude  PSBequivalent=0
  Conn1 : PMIOPort  Port=1  Side=Left
  Conn2 : PMIOPort  Port=2  Side=Left
  wires:
  V_Load1/1 -> Relational Operator/1
  Constant1/1 -> Relational Operator/2
  Detect Rise Positive/1 -> Switch1/2
  Constant3/1 -> Switch1/3
  Relational Operator/1 -> Detect Rise Positive/1
  Constant2/1 -> Switch1/1
  i_Load/1 -> To Workspace1/1, Scope1/1
  V_Load/1 -> To Workspace4/1, Scope/1
  Switch1/1 -> Thyristor/1
  connections:
  Series RLC Branch1/LConn1 -- Series RLC Branch/RConn1
  Series RLC Branch/LConn1 -- V_Load/LConn1 -- Thyristor/RConn1
  V_Load/LConn2 -- Ground2/LConn1 -- Series RLC Branch1/RConn1
  i_Load/RConn1 -- Thyristor/LConn1
  V_Load1/LConn1 -- i_Load/LConn1 -- Conn1/RConn1
  V_Load1/LConn2 -- Conn2/RConn1

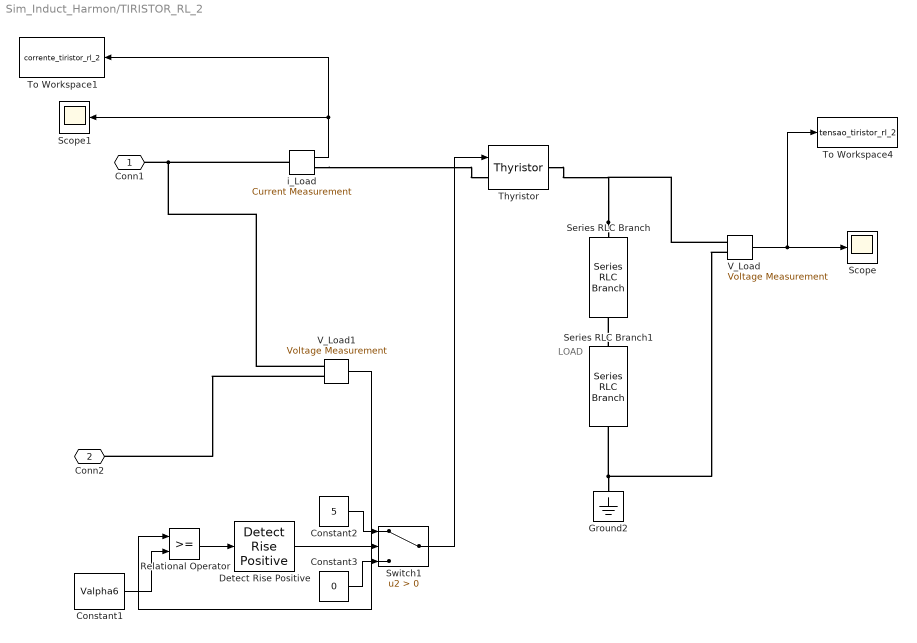
== system Sim_Induct_Harmon/TIRISTOR_RL_2 ==
  note: LOAD
  Constant1 : Constant  Value=Valpha6
  Constant2 : Constant  Value=5
  Constant3 : Constant  Value=0
  Detect Rise Positive : simulink/Logic and Bit Operations/Detect Rise Positive  vinit=0  OutDataTypeStr=boolean
  Ground2 : powerlib/Elements/Ground  LConnTagsString=a
  Relational Operator : RelationalOperator  OutDataTypeStr=boolean  RndMeth=Simplest
  Scope : Scope
  Scope1 : Scope
  Series RLC Branch : powerlib/Elements/Series RLC Branch  LConnTagsString=__new0  RConnTagsString=__new0  BranchType=R  Resistance=R62  Inductance=1e-3  SetiL0=off  InitialCurrent=0  Capacitance=1e-6  Setx0=off  InitialVoltage=0  Measurements=None
  Series RLC Branch1 : powerlib/Elements/Series RLC Branch  LConnTagsString=__new0  RConnTagsString=__new0  BranchType=L  Resistance=1  Inductance=L62  SetiL0=off  InitialCurrent=0  Capacitance=1e-6  Setx0=off  InitialVoltage=0  Measurements=None
  Switch1 : Switch  Criteria=u2 > Threshold
  Thyristor : powerlib/Power Electronics/Thyristor  Ron=0.001  Lon=0  Vf=0.8  IC=0  Rs=500  Cs=250e-9  Measurements=off
  To Workspace1 : ToWorkspace  VariableName=corrente_tiristor_rl_2  SampleTime=-1
  To Workspace4 : ToWorkspace  VariableName=tensao_tiristor_rl_2  SampleTime=-1
  V_Load : powerlib/Measurements/Voltage Measurement  PhasorSimulation=off  OutputType=Complex  PSBequivalent=0
  V_Load1 : powerlib/Measurements/Voltage Measurement  PhasorSimulation=off  OutputType=Complex  PSBequivalent=0
  i_Load : powerlib/Measurements/Current Measurement  Tag=PoWeRsYsTeMmEaSuReMeNt  PhasorSimulation=off  OutputType=Magnitude  PSBequivalent=0
  Conn1 : PMIOPort  Port=1  Side=Left
  Conn2 : PMIOPort  Port=2  Side=Left
  wires:
  V_Load1/1 -> Relational Operator/1
  Constant1/1 -> Relational Operator/2
  Detect Rise Positive/1 -> Switch1/2
  Constant3/1 -> Switch1/3
  Relational Operator/1 -> Detect Rise Positive/1
  Constant2/1 -> Switch1/1
  i_Load/1 -> To Workspace1/1, Scope1/1
  V_Load/1 -> To Workspace4/1, Scope/1
  Switch1/1 -> Thyristor/1
  connections:
  Series RLC Branch1/LConn1 -- Series RLC Branch/RConn1
  Series RLC Branch/LConn1 -- V_Load/LConn1 -- Thyristor/RConn1
  V_Load/LConn2 -- Ground2/LConn1 -- Series RLC Branch1/RConn1
  i_Load/RConn1 -- Thyristor/LConn1
  V_Load1/LConn1 -- i_Load/LConn1 -- Conn1/RConn1
  V_Load1/LConn2 -- Conn2/RConn1

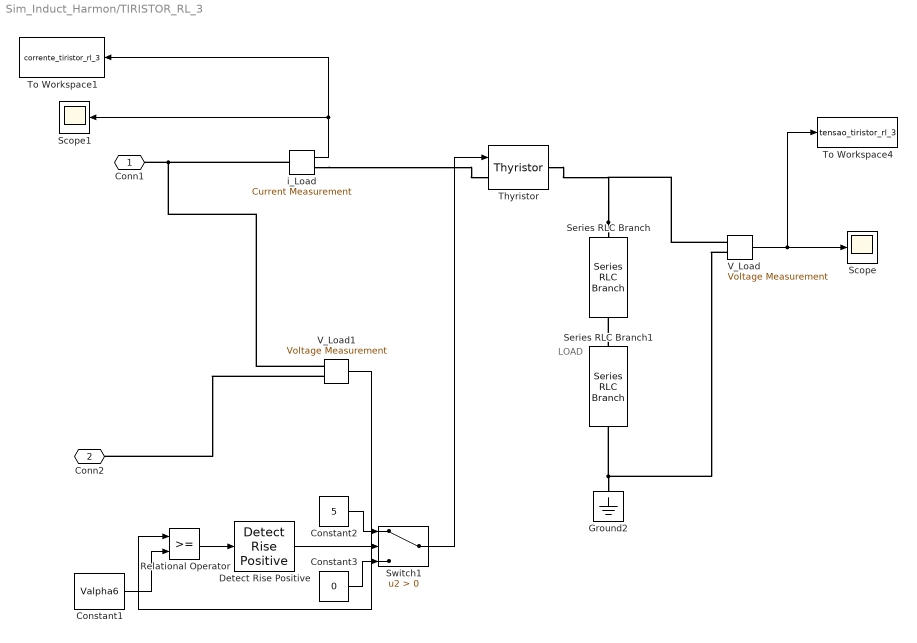
== system Sim_Induct_Harmon/TIRISTOR_RL_3 ==
  note: LOAD
  Constant1 : Constant  Value=Valpha6
  Constant2 : Constant  Value=5
  Constant3 : Constant  Value=0
  Detect Rise Positive : simulink/Logic and Bit Operations/Detect Rise Positive  vinit=0  OutDataTypeStr=boolean
  Ground2 : powerlib/Elements/Ground  LConnTagsString=a
  Relational Operator : RelationalOperator  OutDataTypeStr=boolean  RndMeth=Simplest
  Scope : Scope
  Scope1 : Scope
  Series RLC Branch : powerlib/Elements/Series RLC Branch  LConnTagsString=__new0  RConnTagsString=__new0  BranchType=R  Resistance=R63  Inductance=1e-3  SetiL0=off  InitialCurrent=0  Capacitance=1e-6  Setx0=off  InitialVoltage=0  Measurements=None
  Series RLC Branch1 : powerlib/Elements/Series RLC Branch  LConnTagsString=__new0  RConnTagsString=__new0  BranchType=L  Resistance=1  Inductance=L63  SetiL0=off  InitialCurrent=0  Capacitance=1e-6  Setx0=off  InitialVoltage=0  Measurements=None
  Switch1 : Switch  Criteria=u2 > Threshold
  Thyristor : powerlib/Power Electronics/Thyristor  Ron=0.001  Lon=0  Vf=0.8  IC=0  Rs=500  Cs=250e-9  Measurements=off
  To Workspace1 : ToWorkspace  VariableName=corrente_tiristor_rl_3  SampleTime=-1
  To Workspace4 : ToWorkspace  VariableName=tensao_tiristor_rl_3  SampleTime=-1
  V_Load : powerlib/Measurements/Voltage Measurement  PhasorSimulation=off  OutputType=Complex  PSBequivalent=0
  V_Load1 : powerlib/Measurements/Voltage Measurement  PhasorSimulation=off  OutputType=Complex  PSBequivalent=0
  i_Load : powerlib/Measurements/Current Measurement  Tag=PoWeRsYsTeMmEaSuReMeNt  PhasorSimulation=off  OutputType=Magnitude  PSBequivalent=0
  Conn1 : PMIOPort  Port=1  Side=Left
  Conn2 : PMIOPort  Port=2  Side=Left
  wires:
  V_Load1/1 -> Relational Operator/1
  Constant1/1 -> Relational Operator/2
  Detect Rise Positive/1 -> Switch1/2
  Constant3/1 -> Switch1/3
  Relational Operator/1 -> Detect Rise Positive/1
  Constant2/1 -> Switch1/1
  i_Load/1 -> To Workspace1/1, Scope1/1
  V_Load/1 -> To Workspace4/1, Scope/1
  Switch1/1 -> Thyristor/1
  connections:
  Series RLC Branch1/LConn1 -- Series RLC Branch/RConn1
  Series RLC Branch/LConn1 -- V_Load/LConn1 -- Thyristor/RConn1
  V_Load/LConn2 -- Ground2/LConn1 -- Series RLC Branch1/RConn1
  i_Load/RConn1 -- Thyristor/LConn1
  V_Load1/LConn1 -- i_Load/LConn1 -- Conn1/RConn1
  V_Load1/LConn2 -- Conn2/RConn1

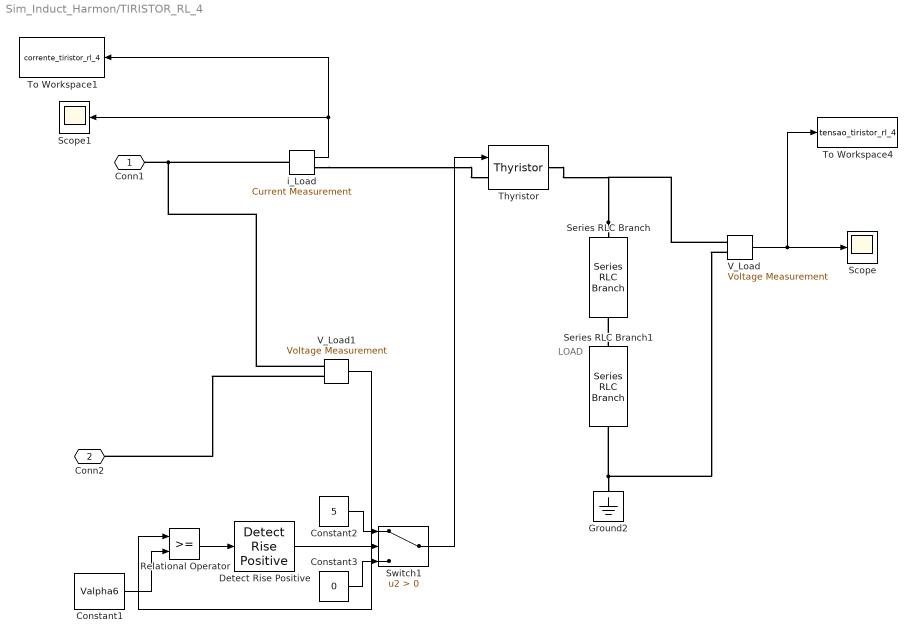
== system Sim_Induct_Harmon/TIRISTOR_RL_4 ==
  note: LOAD
  Constant1 : Constant  Value=Valpha6
  Constant2 : Constant  Value=5
  Constant3 : Constant  Value=0
  Detect Rise Positive : simulink/Logic and Bit Operations/Detect Rise Positive  vinit=0  OutDataTypeStr=boolean
  Ground2 : powerlib/Elements/Ground  LConnTagsString=a
  Relational Operator : RelationalOperator  OutDataTypeStr=boolean  RndMeth=Simplest
  Scope : Scope
  Scope1 : Scope
  Series RLC Branch : powerlib/Elements/Series RLC Branch  LConnTagsString=__new0  RConnTagsString=__new0  BranchType=R  Resistance=R64  Inductance=1e-3  SetiL0=off  InitialCurrent=0  Capacitance=1e-6  Setx0=off  InitialVoltage=0  Measurements=None
  Series RLC Branch1 : powerlib/Elements/Series RLC Branch  LConnTagsString=__new0  RConnTagsString=__new0  BranchType=L  Resistance=1  Inductance=L64  SetiL0=off  InitialCurrent=0  Capacitance=1e-6  Setx0=off  InitialVoltage=0  Measurements=None
  Switch1 : Switch  Criteria=u2 > Threshold
  Thyristor : powerlib/Power Electronics/Thyristor  Ron=0.001  Lon=0  Vf=0.8  IC=0  Rs=500  Cs=250e-9  Measurements=off
  To Workspace1 : ToWorkspace  VariableName=corrente_tiristor_rl_4  SampleTime=-1
  To Workspace4 : ToWorkspace  VariableName=tensao_tiristor_rl_4  SampleTime=-1
  V_Load : powerlib/Measurements/Voltage Measurement  PhasorSimulation=off  OutputType=Complex  PSBequivalent=0
  V_Load1 : powerlib/Measurements/Voltage Measurement  PhasorSimulation=off  OutputType=Complex  PSBequivalent=0
  i_Load : powerlib/Measurements/Current Measurement  Tag=PoWeRsYsTeMmEaSuReMeNt  PhasorSimulation=off  OutputType=Magnitude  PSBequivalent=0
  Conn1 : PMIOPort  Port=1  Side=Left
  Conn2 : PMIOPort  Port=2  Side=Left
  wires:
  V_Load1/1 -> Relational Operator/1
  Constant1/1 -> Relational Operator/2
  Detect Rise Positive/1 -> Switch1/2
  Constant3/1 -> Switch1/3
  Relational Operator/1 -> Detect Rise Positive/1
  Constant2/1 -> Switch1/1
  i_Load/1 -> To Workspace1/1, Scope1/1
  V_Load/1 -> To Workspace4/1, Scope/1
  Switch1/1 -> Thyristor/1
  connections:
  Series RLC Branch1/LConn1 -- Series RLC Branch/RConn1
  Series RLC Branch/LConn1 -- V_Load/LConn1 -- Thyristor/RConn1
  V_Load/LConn2 -- Ground2/LConn1 -- Series RLC Branch1/RConn1
  i_Load/RConn1 -- Thyristor/LConn1
  V_Load1/LConn1 -- i_Load/LConn1 -- Conn1/RConn1
  V_Load1/LConn2 -- Conn2/RConn1

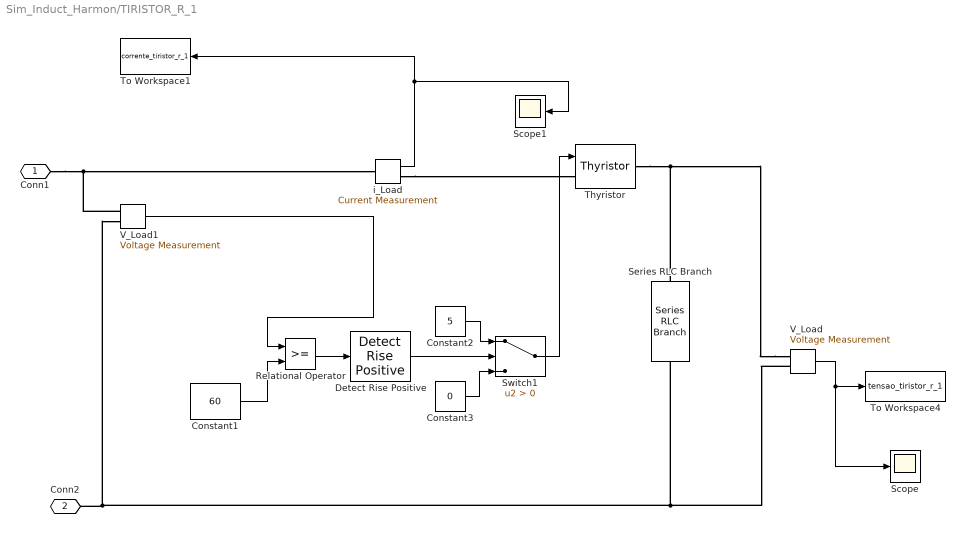
== system Sim_Induct_Harmon/TIRISTOR_R_1 ==
  Constant1 : Constant  Value=60
  Constant2 : Constant  Value=5
  Constant3 : Constant  Value=0
  Detect Rise Positive : simulink/Logic and Bit Operations/Detect Rise Positive  vinit=0  OutDataTypeStr=boolean
  Relational Operator : RelationalOperator  OutDataTypeStr=boolean  RndMeth=Simplest
  Scope : Scope
  Scope1 : Scope
  Series RLC Branch : powerlib/Elements/Series RLC Branch  LConnTagsString=__new0  RConnTagsString=__new0  BranchType=R  Resistance=R51  Inductance=1e-3  SetiL0=off  InitialCurrent=0  Capacitance=1e-6  Setx0=off  InitialVoltage=0  Measurements=None
  Switch1 : Switch  Criteria=u2 > Threshold
  Thyristor : powerlib/Power Electronics/Thyristor  Ron=0.001  Lon=0  Vf=0.8  IC=0  Rs=500  Cs=250e-9  Measurements=off
  To Workspace1 : ToWorkspace  VariableName=corrente_tiristor_r_1  SampleTime=-1
  To Workspace4 : ToWorkspace  VariableName=tensao_tiristor_r_1  SampleTime=-1
  V_Load : powerlib/Measurements/Voltage Measurement  PhasorSimulation=off  OutputType=Complex  PSBequivalent=0
  V_Load1 : powerlib/Measurements/Voltage Measurement  PhasorSimulation=off  OutputType=Complex  PSBequivalent=0
  i_Load : powerlib/Measurements/Current Measurement  Tag=PoWeRsYsTeMmEaSuReMeNt  PhasorSimulation=off  OutputType=Magnitude  PSBequivalent=0
  Conn1 : PMIOPort  Port=1  Side=Left
  Conn2 : PMIOPort  Port=2  Side=Left
  wires:
  Constant3/1 -> Switch1/3
  Constant2/1 -> Switch1/1
  Constant1/1 -> Relational Operator/2
  Relational Operator/1 -> Detect Rise Positive/1
  i_Load/1 -> To Workspace1/1, Scope1/1
  Detect Rise Positive/1 -> Switch1/2
  V_Load1/1 -> Relational Operator/1
  V_Load/1 -> Scope/1, To Workspace4/1
  Switch1/1 -> Thyristor/1
  connections:
  V_Load/LConn1 -- Series RLC Branch/LConn1 -- Thyristor/RConn1
  Conn1/RConn1 -- V_Load1/LConn1 -- i_Load/LConn1
  i_Load/RConn1 -- Thyristor/LConn1
  V_Load/LConn2 -- Series RLC Branch/RConn1 -- Conn2/RConn1 -- V_Load1/LConn2

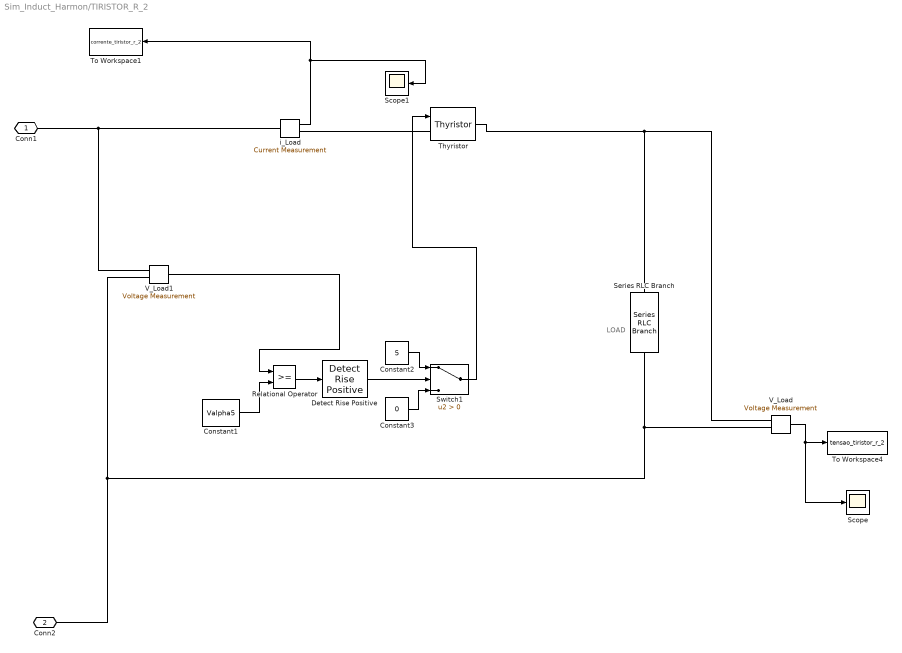
== system Sim_Induct_Harmon/TIRISTOR_R_2 ==
  note: LOAD
  Constant1 : Constant  Value=Valpha5
  Constant2 : Constant  Value=5
  Constant3 : Constant  Value=0
  Detect Rise Positive : simulink/Logic and Bit Operations/Detect Rise Positive  vinit=0  OutDataTypeStr=boolean
  Relational Operator : RelationalOperator  OutDataTypeStr=boolean  RndMeth=Simplest
  Scope : Scope
  Scope1 : Scope
  Series RLC Branch : powerlib/Elements/Series RLC Branch  LConnTagsString=__new0  RConnTagsString=__new0  BranchType=R  Resistance=R52  Inductance=1e-3  SetiL0=off  InitialCurrent=0  Capacitance=1e-6  Setx0=off  InitialVoltage=0  Measurements=None
  Switch1 : Switch  Criteria=u2 > Threshold
  Thyristor : powerlib/Power Electronics/Thyristor  Ron=0.001  Lon=0  Vf=0.8  IC=0  Rs=500  Cs=250e-9  Measurements=off
  To Workspace1 : ToWorkspace  VariableName=corrente_tiristor_r_2  SampleTime=-1
  To Workspace4 : ToWorkspace  VariableName=tensao_tiristor_r_2  SampleTime=-1
  V_Load : powerlib/Measurements/Voltage Measurement  PhasorSimulation=off  OutputType=Complex  PSBequivalent=0
  V_Load1 : powerlib/Measurements/Voltage Measurement  PhasorSimulation=off  OutputType=Complex  PSBequivalent=0
  i_Load : powerlib/Measurements/Current Measurement  Tag=PoWeRsYsTeMmEaSuReMeNt  PhasorSimulation=off  OutputType=Magnitude  PSBequivalent=0
  Conn1 : PMIOPort  Port=1  Side=Left
  Conn2 : PMIOPort  Port=2  Side=Left
  wires:
  Constant3/1 -> Switch1/3
  Constant2/1 -> Switch1/1
  Constant1/1 -> Relational Operator/2
  Relational Operator/1 -> Detect Rise Positive/1
  i_Load/1 -> To Workspace1/1, Scope1/1
  Detect Rise Positive/1 -> Switch1/2
  V_Load1/1 -> Relational Operator/1
  V_Load/1 -> Scope/1, To Workspace4/1
  Switch1/1 -> Thyristor/1
  connections:
  V_Load/LConn1 -- Thyristor/RConn1 -- Series RLC Branch/LConn1
  Conn1/RConn1 -- V_Load1/LConn1 -- i_Load/LConn1
  i_Load/RConn1 -- Thyristor/LConn1
  V_Load/LConn2 -- Series RLC Branch/RConn1 -- Conn2/RConn1 -- V_Load1/LConn2

== system Sim_Induct_Harmon/TIRISTOR_R_3 ==
  note: LOAD
  Constant1 : Constant  Value=Valpha5
  Constant2 : Constant  Value=5
  Constant3 : Constant  Value=0
  Detect Rise Positive : simulink/Logic and Bit Operations/Detect Rise Positive  vinit=0  OutDataTypeStr=boolean
  Relational Operator : RelationalOperator  OutDataTypeStr=boolean  RndMeth=Simplest
  Scope : Scope
  Scope1 : Scope
  Series RLC Branch : powerlib/Elements/Series RLC Branch  LConnTagsString=__new0  RConnTagsString=__new0  BranchType=R  Resistance=R53  Inductance=1e-3  SetiL0=off  InitialCurrent=0  Capacitance=1e-6  Setx0=off  InitialVoltage=0  Measurements=None
  Switch1 : Switch  Criteria=u2 > Threshold
  Thyristor : powerlib/Power Electronics/Thyristor  Ron=0.001  Lon=0  Vf=0.8  IC=0  Rs=500  Cs=250e-9  Measurements=off
  To Workspace1 : ToWorkspace  VariableName=corrente_tiristor_r_3  SampleTime=-1
  To Workspace4 : ToWorkspace  VariableName=tensao_tiristor_r_3  SampleTime=-1
  V_Load : powerlib/Measurements/Voltage Measurement  PhasorSimulation=off  OutputType=Complex  PSBequivalent=0
  V_Load1 : powerlib/Measurements/Voltage Measurement  PhasorSimulation=off  OutputType=Complex  PSBequivalent=0
  i_Load : powerlib/Measurements/Current Measurement  Tag=PoWeRsYsTeMmEaSuReMeNt  PhasorSimulation=off  OutputType=Magnitude  PSBequivalent=0
  Conn1 : PMIOPort  Port=1  Side=Left
  Conn2 : PMIOPort  Port=2  Side=Left
  wires:
  Constant3/1 -> Switch1/3
  Constant2/1 -> Switch1/1
  Constant1/1 -> Relational Operator/2
  Relational Operator/1 -> Detect Rise Positive/1
  i_Load/1 -> To Workspace1/1, Scope1/1
  Detect Rise Positive/1 -> Switch1/2
  V_Load1/1 -> Relational Operator/1
  V_Load/1 -> Scope/1, To Workspace4/1
  Switch1/1 -> Thyristor/1
  connections:
  V_Load/LConn1 -- Thyristor/RConn1 -- Series RLC Branch/LConn1
  Conn1/RConn1 -- V_Load1/LConn1 -- i_Load/LConn1
  i_Load/RConn1 -- Thyristor/LConn1
  V_Load/LConn2 -- Series RLC Branch/RConn1 -- Conn2/RConn1 -- V_Load1/LConn2

== system Sim_Induct_Harmon/TIRISTOR_R_4 ==
  note: LOAD
  Constant1 : Constant  Value=Valpha5
  Constant2 : Constant  Value=5
  Constant3 : Constant  Value=0
  Detect Rise Positive : simulink/Logic and Bit Operations/Detect Rise Positive  vinit=0  OutDataTypeStr=boolean
  Relational Operator : RelationalOperator  OutDataTypeStr=boolean  RndMeth=Simplest
  Scope : Scope
  Scope1 : Scope
  Series RLC Branch : powerlib/Elements/Series RLC Branch  LConnTagsString=__new0  RConnTagsString=__new0  BranchType=R  Resistance=R54  Inductance=1e-3  SetiL0=off  InitialCurrent=0  Capacitance=1e-6  Setx0=off  InitialVoltage=0  Measurements=None
  Switch1 : Switch  Criteria=u2 > Threshold
  Thyristor : powerlib/Power Electronics/Thyristor  Ron=0.001  Lon=0  Vf=0.8  IC=0  Rs=500  Cs=250e-9  Measurements=off
  To Workspace1 : ToWorkspace  VariableName=corrente_tiristor_r_4  SampleTime=-1
  To Workspace4 : ToWorkspace  VariableName=tensao_tiristor_r_4  SampleTime=-1
  V_Load : powerlib/Measurements/Voltage Measurement  PhasorSimulation=off  OutputType=Complex  PSBequivalent=0
  V_Load1 : powerlib/Measurements/Voltage Measurement  PhasorSimulation=off  OutputType=Complex  PSBequivalent=0
  i_Load : powerlib/Measurements/Current Measurement  Tag=PoWeRsYsTeMmEaSuReMeNt  PhasorSimulation=off  OutputType=Magnitude  PSBequivalent=0
  Conn1 : PMIOPort  Port=1  Side=Left
  Conn2 : PMIOPort  Port=2  Side=Left
  wires:
  Constant3/1 -> Switch1/3
  Constant2/1 -> Switch1/1
  Constant1/1 -> Relational Operator/2
  Relational Operator/1 -> Detect Rise Positive/1
  i_Load/1 -> To Workspace1/1, Scope1/1
  Detect Rise Positive/1 -> Switch1/2
  V_Load1/1 -> Relational Operator/1
  V_Load/1 -> Scope/1, To Workspace4/1
  Switch1/1 -> Thyristor/1
  connections:
  V_Load/LConn1 -- Thyristor/RConn1 -- Series RLC Branch/LConn1
  Conn1/RConn1 -- V_Load1/LConn1 -- i_Load/LConn1
  i_Load/RConn1 -- Thyristor/LConn1
  V_Load/LConn2 -- Series RLC Branch/RConn1 -- Conn2/RConn1 -- V_Load1/LConn2

== system Sim_Induct_Harmon/MOTOR_UNIVERSAL_1/Ea_ ==
  in_1 : Inport
  in_2 : Inport  Port=2
  Product : Product  SaturateOnIntegerOverflow=on  RndMeth=Zero  InputSameDT=on  OutDataTypeStr=Inherit: Same as first input
  Sum : Sum  Inputs=+  SaturateOnIntegerOverflow=on  InputSameDT=on  OutDataTypeStr=Inherit: Same as first input
  out_1 : Outport  InitialOutput=0
  wires:
  Sum/1 -> out_1/1
  Product/1 -> Sum/1
  in_1/1 -> Product/1
  in_2/1 -> Product/2

== system Sim_Induct_Harmon/MOTOR_UNIVERSAL_1/Product ==
  in_1 : Inport
  in_2 : Inport  Port=2
  Product : Product  SaturateOnIntegerOverflow=on  RndMeth=Zero  InputSameDT=on  OutDataTypeStr=Inherit: Same as first input
  Sum : Sum  Inputs=+  SaturateOnIntegerOverflow=on  InputSameDT=on  OutDataTypeStr=Inherit: Same as first input
  out_1 : Outport  InitialOutput=0
  wires:
  Sum/1 -> out_1/1
  Product/1 -> Sum/1
  in_1/1 -> Product/1
  in_2/1 -> Product/2

== system Sim_Induct_Harmon/MOTOR_UNIVERSAL_2/Ea_ ==
  in_1 : Inport
  in_2 : Inport  Port=2
  Product : Product  SaturateOnIntegerOverflow=on  RndMeth=Zero  InputSameDT=on  OutDataTypeStr=Inherit: Same as first input
  Sum : Sum  Inputs=+  SaturateOnIntegerOverflow=on  InputSameDT=on  OutDataTypeStr=Inherit: Same as first input
  out_1 : Outport  InitialOutput=0
  wires:
  Sum/1 -> out_1/1
  Product/1 -> Sum/1
  in_1/1 -> Product/1
  in_2/1 -> Product/2

== system Sim_Induct_Harmon/MOTOR_UNIVERSAL_2/Product ==
  in_1 : Inport
  in_2 : Inport  Port=2
  Product : Product  SaturateOnIntegerOverflow=on  RndMeth=Zero  InputSameDT=on  OutDataTypeStr=Inherit: Same as first input
  Sum : Sum  Inputs=+  SaturateOnIntegerOverflow=on  InputSameDT=on  OutDataTypeStr=Inherit: Same as first input
  out_1 : Outport  InitialOutput=0
  wires:
  Sum/1 -> out_1/1
  Product/1 -> Sum/1
  in_1/1 -> Product/1
  in_2/1 -> Product/2
